simulink model "MPC_opt"  (R2020b)
settings: Solver=VariableStepAuto  StartTime=0.0  StopTime=4  RelTol=1e-3
libraries: simulink x1
settings Model: Creator=surya  LastModifiedBy=surya

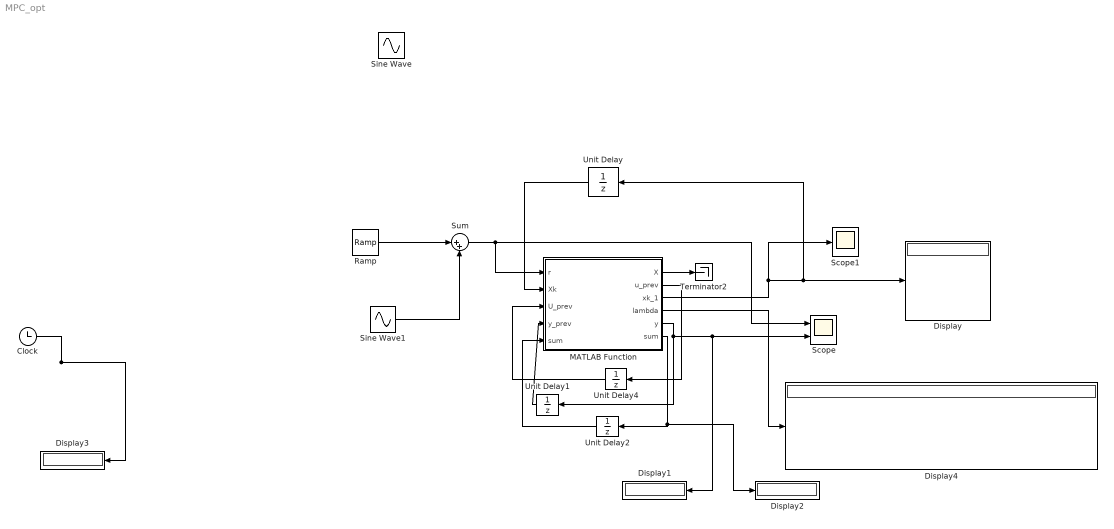
== system MPC_opt ==
  Clock : Clock
      settings: Decimation=1000
  Display{,1..4} (5 alike) : Display
  MATLAB Function : MATLAB Function  TreatAsAtomicUnit=on
  Ramp : simulink/Sources/Ramp  slope=0  start=0  InitialOutput=0.085
  Scope : Scope  NumInputPorts=2
  Scope1 : Scope
  Sine Wave : Sin  Amplitude=500  SampleTime=0
  Sine Wave1 : Sin  Amplitude=0.0008  Frequency=1.5  SampleTime=0
  Sum : Sum  Inputs=|++
  Terminator2 : Terminator
  Unit Delay : UnitDelay  InitialCondition=[0; 0; 0; 0]  SampleTime=-1  HasFrameUpgradeWarning=on
  Unit Delay1 : UnitDelay  SampleTime=-1  HasFrameUpgradeWarning=on
  Unit Delay2 : UnitDelay  SampleTime=-1  HasFrameUpgradeWarning=on
  Unit Delay4 : UnitDelay  SampleTime=-1  HasFrameUpgradeWarning=on
  wires:
  MATLAB Function/1(X) -> Terminator2/1
  Clock/1 -> Display3/1
  MATLAB Function/3(xk_1) -> Unit Delay/1, Display/1, Scope1/1
  Unit Delay/1 -> MATLAB Function/2(Xk)
  MATLAB Function/2(u_prev) -> Unit Delay4/1
  Unit Delay4/1 -> MATLAB Function/3(U_prev)
  MATLAB Function/4(lambda) -> Display4/1
  MATLAB Function/5(y) -> Unit Delay1/1, Scope/2, Display1/1
  Ramp/1 -> Sum/1
  Sine Wave1/1 -> Sum/2
  Sum/1 -> MATLAB Function/1(r), Scope/1
  Unit Delay1/1 -> MATLAB Function/4(y_prev)
  MATLAB Function/6(sum) -> Display2/1, Unit Delay2/1
  Unit Delay2/1 -> MATLAB Function/5("sum ")

== matlab function MPC_opt/MATLAB Function ==
  data: X output; u_prev output; r input; Xk input; xk_1 output; lambda output; U_prev input; y output; y_prev input; sum input; sum output
function [X,u_prev,xk_1,lambda,y,sum] = MPC_opt(r, Xk, U_prev, y_prev, sum)

N = 5;

xk = Xk;  %Perturbed states used in State Space

A = [-1.9311*10^-2 8.8157 -32.17 -0.575; -2.5389*10^-4 -1.0189 0 0.9051; 2.9465*10^-12 0.8223 0 -1.0774; 0 0 1 0];
B = [0.1737; -2.1499; -0.1756; 0];
C = [0 1 0 0];
D = 0;

ref = inv([(A-eye(length(A))) B; C D])*[zeros([length(A),1]);r];
x_r = ref(1:4);
u_r = ref(5);
xr = [x_r;x_r;x_r;x_r;x_r];
ur = u_r*ones([N,1]);

fx = [sign(xk(1)) 0 0 0; 0 sign(xk(2)) 0 0; 0 0 sign(xk(3)) 0; 0 0 0 sign(xk(4))];
Fx = [fx, zeros([4,4]), zeros([4,4]), zeros([4,4]), zeros([4,4]); zeros([4,4]), fx, zeros([4,4]), zeros([4,4]), zeros([4,4]); zeros([4,4]), zeros([4,4]), fx, zeros([4,4]), zeros([4,4]); zeros([4,4]), zeros([4,4]), zeros([4,4]), fx, zeros([4,4]); zeros([4,4]), zeros([4,4]), zeros([4,4]), zeros([4,4]), fx];
Fu = sign(U_prev)*eye(N);   % 8 deg max elevator deflection
bbx = [50*sign(xk(1));0.174*sign(xk(2));0.174*sign(xk(3));0.174*sign(xk(4))];
bx = [bbx;bbx;bbx;bbx;bbx];
bu = 0.0873*ones([N,1])*sign(U_prev);

A_c = [A;A^2;A^3;A^4;A^5];
B_c = [B zeros([4,1]) zeros([4,1]) zeros([4,1]) zeros([4,1]); A*B B zeros([4,1]) zeros([4,1]) zeros([4,1]); A^2*B A*B B zeros([4,1]) zeros([4,1]); A^3*B A^2*B A*B B zeros([4,1]); A^4*B A^3*B A^2*B A*B B];

Q = [2*10^3 0 0 0; 0 2*10^3 0 0; 0 0 2*10^3 0; 0 0 0 2*10^5];
R = 2*10^2;
P = [2*10^4 0 0 0; 0 2*10^4 0 0; 0 0 2*10^4 0; 0 0 0 2*10^4 ];
Q_c = [Q zeros([4,4]) zeros([4,4]) zeros([4,4]) zeros([4,4]); zeros([4,4]) Q zeros([4,4]) zeros([4,4]) zeros([4,4]); zeros([4,4]) zeros([4,4]) Q zeros([4,4]) zeros([4,4]); zeros([4,4]) zeros([4,4]) zeros([4,4]) Q zeros([4,4]); zeros([4,4]) zeros([4,4]) zeros([4,4]) zeros([4,4]) P];
R_c = R*eye(N);
M = [Fu; Fx*B_c];
L = [bu; (bx-Fx*A_c*xk)];
J = -0.0135;

lambda = -inv(eye(length(M*inv(B_c'*Q_c*B_c + R_c)*M')) + 0.5*M*inv(B_c'*Q_c*B_c + R_c)*M')*(M*inv(B_c'*Q_c*B_c + R_c)*(B_c'*Q_c*A_c*xk - B_c'*Q_c*xr - R_c'*ur) + L);
U_opt = -inv(B_c'*Q_c*B_c + R_c)*(B_c'*Q_c*A_c*xk - B_c'*Q_c*xr - R_c'*ur + 0.5*M'*lambda);
e = r-y_prev;
X = A_c*xk + B_c*U_opt;
if sign(e)*e < 2*10^-3*sign(e)
    sum = sum + e;
    det_u = J*sum;
else
    det_u = 0;
end
xk_1 = A*xk + B*(U_opt(1)+det_u);
y = C*xk;
u_prev = U_opt(N)+det_u;

end
